simulink model "BPSK_music"  (R2021b)
settings: Solver=VariableStepAuto  StartTime=0.0  StopTime=13.5  RelTol=1e-3
libraries: commdigbbndpm3 x2, commutil2 x2, commchan3 x1, dspsnks4 x1, commsink2 x1, dspvision x1
settings Model: Creator=PC  LastModifiedBy=PC

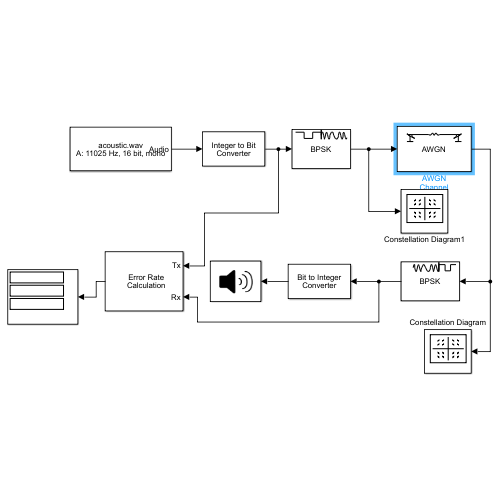
[thumbnail: Simulink's stored preview of the top-level diagram]
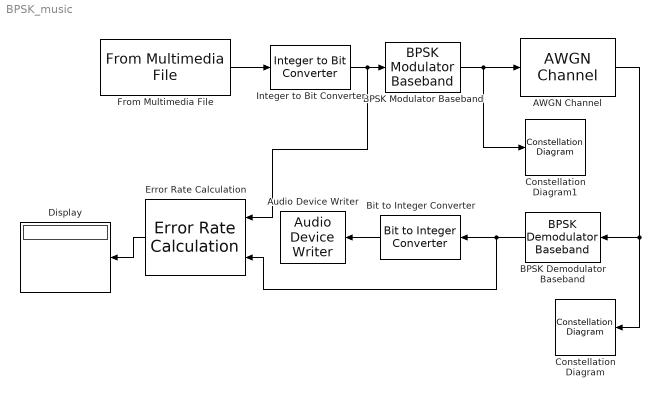
== system BPSK_music ==
  AWGN Channel : commchan3/AWGN Channel  InputProcessing=Columns as channels (frame based)  seed=67  noiseMode="Signal to noise ratio  (SNR)"  EbNodB=1  EsNodB=10  SNRdB=0  bitsPerSym=1  Ps=1  Tsym=1  variance=1
  Audio Device Writer : dspsnks4/Audio Device Writer  Driver=DirectSound  Device=Default  InheritSampleRate=on  SampleRate=44100  BitDepth=16-bit integer  BufferSize=4096  NumBuffers=10  DefaultOutputChannelMapping=on  OutputChannelMapping=1:2  OutputNumUnderrunSamples=off  DriverIdx=1  DeviceWarnFlag=''
  BPSK Demodulator Baseband : commdigbbndpm3/BPSK Demodulator Baseband  DecType=Hard decision  VarSource=Dialog  Variance=1  Ph=0  outDtype=Inherit via internal rule  derotateFactorWordLen=16  derotateFactorDataTypeStr=Inherit: Same word length as input  derotateFactorLastDataTypeStr=Inherit: Same word length as input
  BPSK Modulator Baseband : commdigbbndpm3/BPSK Modulator Baseband  Ph=0  outDtype=double  outWordLen=16  outUDDataType=sfix(16)  outFracLenMode=Best precision  outFracLen=15  outDataTypeStr=double  outLastDataTypeStr=double
  Bit to Integer Converter : commutil2/Bit to Integer Converter  nbits=16  bitOrder=MSB first  signedOutputValues=Unsigned  outDtype=int16  outDtypeSigned=Inherit via internal rule
  Constellation Diagram : ConstellationDiagram
  Constellation Diagram1 : ConstellationDiagram
  Display : Display
  Error Rate Calculation : commsink2/Error Rate Calculation  N=0  st_delay=0  cp_mode=Entire frame  subframe=[]  PMode=Port  WsName=ErrorVec  RsMode2=off  stop=off  numErr=100  maxBits=1e6
  From Multimedia File : dspvision/From Multimedia File  inputFilename=C:\Users\PC\Documents\MATLAB\acoustic.wav  readRange=[1 Inf]  loop=on  numPlays=inf  outputStreams=Audio only  videoDataType=single  audioDataType=double  inheritSampleTime=on  userDefinedSampleTime=1/30  noAudioOutput=off  isIntensityVideo=off  fourcc=RGB  colorVideoFormat=Separate color signals  outputEOF=off  dataOrg=Column-major  audioFrameSize=1024  computeAudioFrameSize=off  outSamplingMode=Sample based
  Integer to Bit Converter : commutil2/Integer to Bit Converter  nbits=16  signedInputValues=Signed  bitOrder=MSB first  outDtype=double
  wires:
  BPSK Modulator Baseband/1 -> Constellation Diagram1/1, AWGN Channel/1
  AWGN Channel/1 -> Constellation Diagram/1, BPSK Demodulator Baseband/1
  Integer to Bit Converter/1 -> Error Rate Calculation/1, BPSK Modulator Baseband/1
  BPSK Demodulator Baseband/1 -> Error Rate Calculation/2, Bit to Integer Converter/1
  Bit to Integer Converter/1 -> Audio Device Writer/1
  From Multimedia File/1 -> Integer to Bit Converter/1
  Error Rate Calculation/1 -> Display/1
